simulink model "QAM64"  (R2015a)
settings: Solver=ode45  StartTime=0.0  StopTime=10.0  RelTol=1e-3
libraries: commdigbbndam3 x2, commchan3 x1, commsink2 x1, commrandsrc2 x1
settings Model: Creator=Lenovo  LastModifiedBy=Lenovo

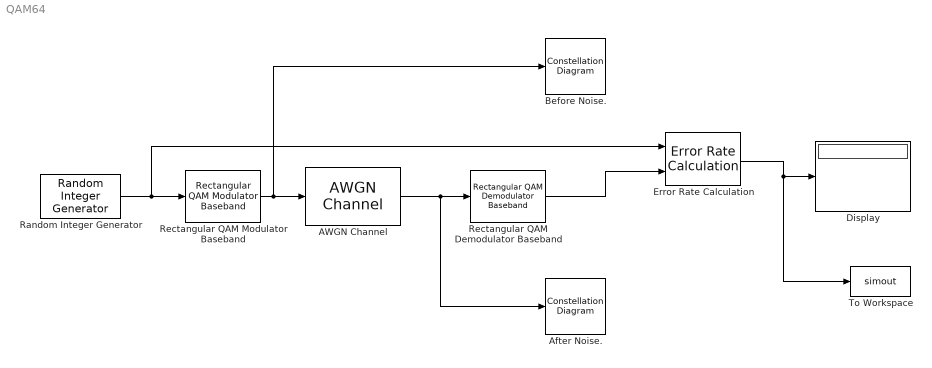
== system QAM64 ==
  AWGN Channel : commchan3/AWGN Channel  InputProcessing=Columns as channels (frame based)  seed=67  noiseMode="Signal to noise ratio  (Eb/No)"  EbNodB=EbNo  EsNodB=10  SNRdB=10  bitsPerSym=1  Ps=1  Tsym=1  variance=1
  "After Noise. " : ConstellationDiagram
  Before Noise. : ConstellationDiagram
  Display : Display
  Error Rate Calculation : commsink2/Error Rate Calculation  N=0  st_delay=0  cp_mode=Entire frame  subframe=[]  PMode=Port  WsName=ErrorVec  RsMode2=off  stop=on  numErr=maxNumErrs  maxBits=maxNumBits
  Random Integer Generator : commrandsrc2/Random Integer Generator  mul=64  seed=37  Ts=1  frameBased=on  sampPerFrame=100  orient=off  outDataType=double
  Rectangular QAM Demodulator Baseband : commdigbbndam3/Rectangular QAM Demodulator Baseband  M=64  PowType=Min. distance between symbols  MinDist=2  AvgPow=1000000  PeakPow=1  Ph=0  Dec=Binary  Mapping=[0:15]  OutType=Integer  DecType=Hard decision  VarSource=Dialog  Variance=1  outDtype1=Inherit via internal rule  outDtype2=Inherit via internal rule  derotateFactorWordLen=16  denormFactorWordLen=16  prodOutWordLen=32  prodOutRoundingMode=Floor  prodOutOverflowMode=Wrap  sumWordLen=32
  Rectangular QAM Modulator Baseband : commdigbbndam3/Rectangular QAM Modulator Baseband  M=64  InType=Integer  Enc=Binary  Mapping=[0:15]  PowType=Min. distance between symbols  MinDist=2  AvgPow=1000000  PeakPow=1  Ph=0  outDtype=double  outWordLen=16  outUDDataType=sfix(16)  outFracLenMode=Best precision  outFracLen=15
  To Workspace : ToWorkspace  VariableName=simout  SampleTime=-1
      settings: Save2DSignal=2-D array (concatenate along first dimension)
  wires:
  Error Rate Calculation/1 -> Display/1, To Workspace/1
  Random Integer Generator/1 -> Rectangular QAM Modulator Baseband/1, Error Rate Calculation/1
  AWGN Channel/1 -> Rectangular QAM Demodulator Baseband/1, "After Noise. "/1
  Rectangular QAM Modulator Baseband/1 -> AWGN Channel/1, Before Noise./1
  Rectangular QAM Demodulator Baseband/1 -> Error Rate Calculation/2
